simulink model "untitled"  (R2020b)
settings: Solver=VariableStepAuto  StartTime=0.0  StopTime=500  RelTol=1e-3
values from neighbouring files (symbols this model uses):
  dt = random('LogNormal',0,0.432,1,1)    [m.m]
undefined symbols (not defined in the file or in its folder): m, n
settings Model: Creator=73561  LastModifiedBy=73561

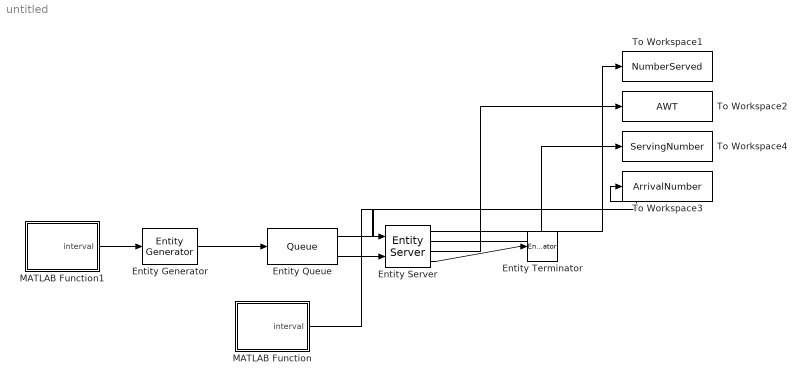
== system untitled ==
  Entity Generator : EntityGenerator  OutputPortMessageModes=m  TimeSource=Signal port  Period=dt  IntergenerationTimeAction=|  AttributeName=Attribute1|data1|data2  AttributeInitialValue=1|2|3  EntityType=Structured  EntityTypeName=Entity
      | %dt = random('LogNormal',0,0.432,1,1);
      | %rng(3,'twister');
      | dt = lognrnd(0, 0.432);
      settings: InputPortMap=u1
  Entity Queue : Queue  InputPortMessageModes=m  OutputPortMessageModes=n,m  Capacity=10000  NumberEntitiesDeparted=on
      settings: OutputPortMap=o0,o5
  Entity Server : EntityServer  InputPortMessageModes=n,m  OutputPortMessageModes=n,n,n,m  Capacity=99999  ServiceTimeSource=Signal port  ServiceTimeAction=dt = random('wbl',79.29,1.077)+256.3485  NumberEntitiesDeparted=on  NumberEntitiesInBlock=on  AverageWait=on
      settings: InputPortMap=u0,u2  OutputPortMap=o0,o1,o4,o9
  Entity Terminator : EntityTerminator  InputPortMessageModes=m
  MATLAB Function : MATLAB Function  TreatAsAtomicUnit=on
  MATLAB Function1 : MATLAB Function  TreatAsAtomicUnit=on
  To Workspace1 : ToWorkspace  VariableName=NumberServed  SaveFormat=Timeseries  SampleTime=-1
  To Workspace2 : ToWorkspace  VariableName=AWT  SaveFormat=Timeseries  SampleTime=-1
  To Workspace3 : ToWorkspace  VariableName=ArrivalNumber  SaveFormat=Timeseries  SampleTime=-1
  To Workspace4 : ToWorkspace  VariableName=ServingNumber  SaveFormat=Timeseries  SampleTime=-1
  wires:
  Entity Generator/1 -> Entity Queue/1
  Entity Queue/2 -> Entity Server/2
  Entity Server/4 -> Entity Terminator/1
  MATLAB Function/1(interval) -> Entity Server/1
  Entity Server/1 -> To Workspace1/1
  Entity Server/3 -> To Workspace2/1
  Entity Server/2 -> To Workspace4/1
  Entity Queue/1 -> To Workspace3/1
  MATLAB Function1/1(interval) -> Entity Generator/1

== matlab function untitled/MATLAB Function ==
  data: interval output
function interval = generateArrivalInterval()
    persistent idx  % 保持随机数序列的索引位置
    persistent comb % 保存随机数序列
    
    if isempty(idx)  % 如果索引为空，则生成随机数序列
        dtser1 = random('wbl', 54.26, 1.12, 50000, 1) + 182.31;
        dtser2 = -random('wbl', 54.26, 1.12, 50000, 1) + 182.31;
        comb = vertcat(dtser1, dtser2);
        comb(comb < 0) = []
        idx = 1;  % 初始化索引位置
    end

    interval = comb(idx);  % 获取当前索引位置的时间间隔
    idx = idx + 1;  % 更新索引位置

    if idx > length(comb)  % 如果索引超出随机数序列长度，则重新开始
        idx = 1;
    end
end

== matlab function untitled/MATLAB Function1 ==
  data: interval output
function interval = generateArrivalInterval()
    persistent idx  % 保持随机数序列的索引位置
    persistent comb % 保存随机数序列
    
    if isempty(idx)  % 如果索引为空，则生成随机数序列
        
        comb = lognrnd(0, 0.432,10000,1)
        idx = 1;  % 初始化索引位置
    end

    interval = comb(idx);  % 获取当前索引位置的时间间隔
    idx = idx + 1;  % 更新索引位置

    if idx > length(comb)  % 如果索引超出随机数序列长度，则重新开始
        idx = 1;
    end
end
